simulink model "train_detection"  (R2024b)
settings: Solver=FixedStepAuto  StartTime=0.0  StopTime=simDuration  FixedStep=0.01  RelTol=1e-3
InitFcn:
  | breakp=[-1, -0.9, -0.8, -0.6, -0.4, -0.2, -0.1, 0, 0.1, 0.2, 0.4, 0.6, 0.8, 1];
  | 
  | splinenew =[-1, -0.92, -0.8, -0.50, -0.28, -0.12, -0.05, 0, 0.005, 0.01, 0.02, 0.025,0.03,0.035];
undefined symbols (not defined in the file or in its folder): Discrete, K, qbreak, Time
libraries: simulink x25, ctrlSharedLib x4, dspfdesign x2
(part 1 of 2)
settings Model: Creator=ARIES  LastModifiedBy=zglin

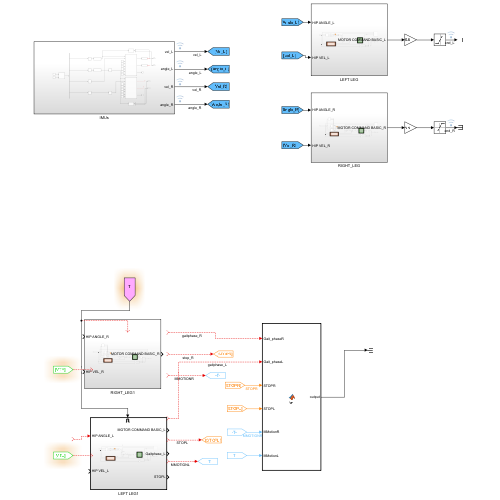
[thumbnail: Simulink's stored preview of the top-level diagram]
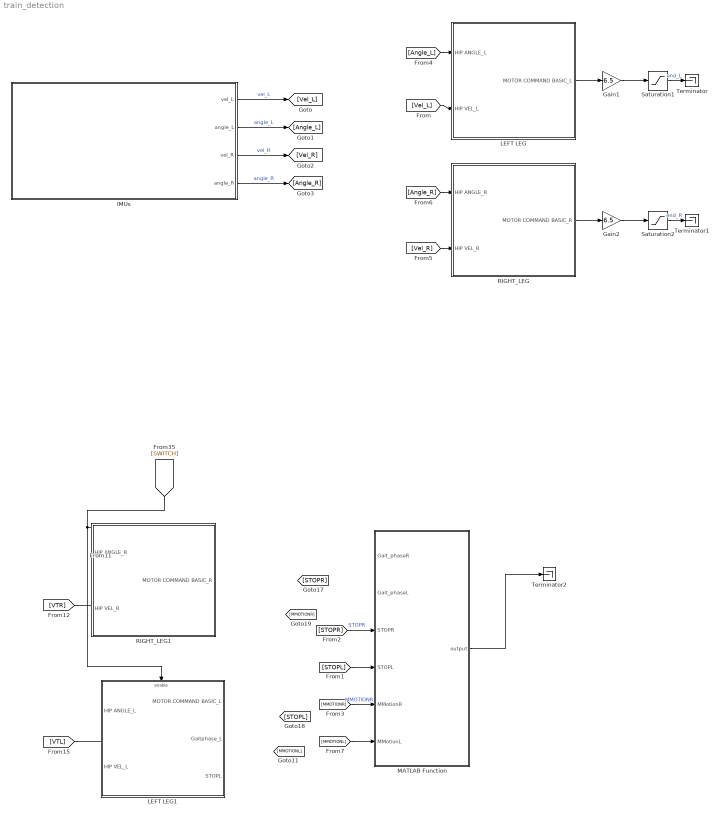
== system train_detection ==
  Gain1 : Gain  Gain=6.5
  Gain2 : Gain  Gain=6.5
  IMUs : Subsystem
  LEFT LEG : Subsystem
  LEFT LEG1 : Subsystem
  MATLAB Function : MATLAB Function  TreatAsAtomicUnit=on
  RIGHT_LEG : Subsystem
  RIGHT_LEG1 : Subsystem
  Saturation1 : Saturate  UpperLimit=900*pi/180  LowerLimit=-900*pi/180
  Saturation2 : Saturate  UpperLimit=900*pi/180  LowerLimit=-900*pi/180
  Terminator : Terminator
  Terminator1 : Terminator
  Terminator2 : Terminator
  wires:
  IMUs/1(vel_L) -> [Vel_L]  "vel_L"
  IMUs/3(vel_R) -> [Vel_R]  "vel_R"
  IMUs/4(angle_R) -> [Angle_R]  "angle_R"
  IMUs/2(angle_L) -> [Angle_L]  "angle_L"
  [Angle_R] -> RIGHT_LEG/1(HIP ANGLE_R)
  RIGHT_LEG/1(MOTOR COMMAND BASIC_R) -> Gain2/1
  [Vel_L] -> LEFT LEG/2(HIP VEL_L)
  [Vel_R] -> RIGHT_LEG/2(HIP VEL_R)
  [Angle_L] -> LEFT LEG/1(HIP ANGLE_L)
  LEFT LEG/1(MOTOR COMMAND BASIC_L) -> Gain1/1
  Gain1/1 -> Saturation1/1
  Gain2/1 -> Saturation2/1
  Saturation1/1 -> Terminator/1  "end_L"
  Saturation2/1 -> Terminator1/1  "end_R"
  ? -> LEFT LEG1/1(HIP ANGLE_L)
  ? -> [STOPR]  "stop_R"
  ? -> [STOPL]  "STOPL"
  [MMOTIONR] -> MATLAB Function/5(MMotionR)  "MMOTIONR"
  [STOPL] -> MATLAB Function/4(STOPL)
  ? -> [MMOTIONL]  "MMOTIONL"
  [MMOTIONL] -> MATLAB Function/6(MMotionL)
  MATLAB Function/1(output) -> Terminator2/1
  ? -> [MMOTIONR]  "MMOTIONR"
  ? -> MATLAB Function/2(Gait_phaseL)  "gaitphase_L"
  [VTL] -> ?
  [SWITCH] -> LEFT LEG1/Enable
  [VTR] -> ?
  ? -> MATLAB Function/1(Gait_phaseR)  "gaitphase_R"
  [STOPR] -> MATLAB Function/3(STOPR)  "STOPR"

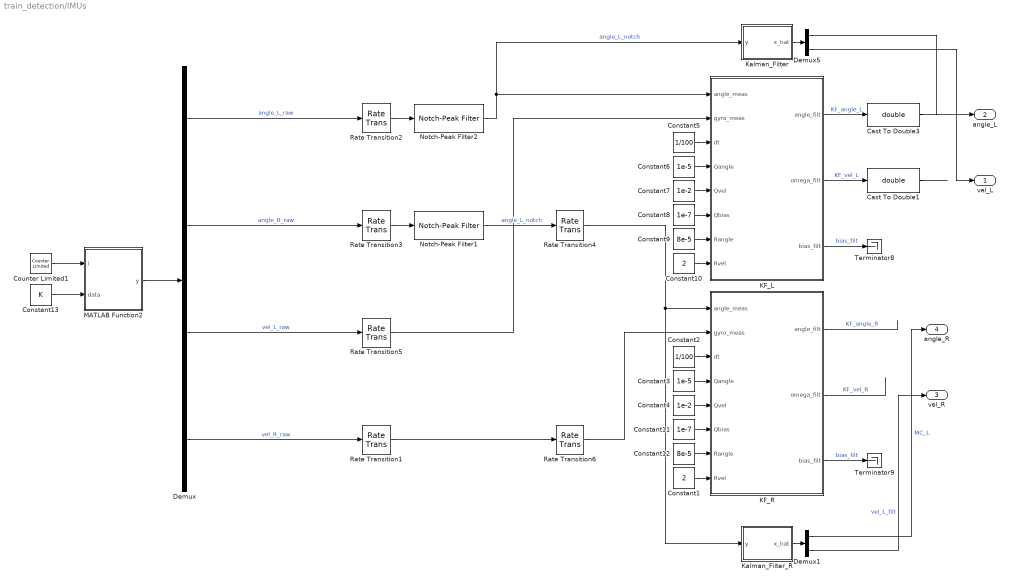
== system train_detection/IMUs ==
  Cast To Double1 : DataTypeConversion  OutDataTypeStr=double  SaturateOnIntegerOverflow=off  RndMeth=Floor
  Cast To Double3 : DataTypeConversion  OutDataTypeStr=double  SaturateOnIntegerOverflow=off  RndMeth=Floor
  Constant1 : Constant  Value=2
  Constant10 : Constant  Value=2
  Constant11 : Constant  Value=1e-7
  Constant12 : Constant  Value=8e-5
  Constant13 : Constant  Value=K
  Constant2 : Constant  Value=1/100
  Constant3 : Constant  Value=1e-5
  Constant4 : Constant  Value=1e-2
  Constant5 : Constant  Value=1/100
  Constant6 : Constant  Value=1e-5
  Constant7 : Constant  Value=1e-2
  Constant8 : Constant  Value=1e-7
  Constant9 : Constant  Value=8e-5
  Counter Limited1 : simulink/Sources/Counter Limited  uplimit=size(K,1)  tsamp=0.01
  Demux : Demux
  Demux1 : Demux  Outputs=2
  Demux5 : Demux  Outputs=2
  KF_L : MATLAB Function  TreatAsAtomicUnit=on  SystemSampleTime=0.01
  KF_R : MATLAB Function  TreatAsAtomicUnit=on  SystemSampleTime=0.01
  Kalman_Filter : MATLAB Function  TreatAsAtomicUnit=on
  Kalman_Filter_R : MATLAB Function  TreatAsAtomicUnit=on
  MATLAB Function2 : MATLAB Function  TreatAsAtomicUnit=on
  Notch-Peak Filter1 : dspfdesign/Notch-Peak Filter  Specification=Bandwidth and center frequency  BandwidthPort=off  Bandwidth=0.1  QualityFactorPort=off  QualityFactor=5  CenterFrequencyPort=off  CenterFrequency=0  BandwidthCoefficientPort=off  BandwidthCoefficient=0.72654  CenterFrequencyCoefficientPort=off  CenterFrequencyCoefficient=0  Output=Notch  SampleRateMode=Specify on dialog  SampleRate=100  SimulateUsing=Interpreted execution
  Notch-Peak Filter2 : dspfdesign/Notch-Peak Filter  Specification=Bandwidth and center frequency  BandwidthPort=off  Bandwidth=0.1  QualityFactorPort=off  QualityFactor=5  CenterFrequencyPort=off  CenterFrequency=0  BandwidthCoefficientPort=off  BandwidthCoefficient=0.72654  CenterFrequencyCoefficientPort=off  CenterFrequencyCoefficient=0  Output=Notch  SampleRateMode=Specify on dialog  SampleRate=100  SimulateUsing=Interpreted execution
  Rate Transition{1..6} (6 alike) : RateTransition  OutPortSampleTime=0.01
  Terminator8 : Terminator
  Terminator9 : Terminator
  vel_L : Outport
  angle_L : Outport  Port=2
  vel_R : Outport  Port=3
  angle_R : Outport  Port=4
  wires:
  Constant1/1 -> KF_R/8(Rvel)
  Counter Limited1/1 -> MATLAB Function2/1(i)
  MATLAB Function2/1(y) -> Demux/1
  Demux5/2 -> vel_L/1
  Demux/1 -> Rate Transition2/1  "angle_L_raw"
  Demux5/1 -> angle_L/1
  Rate Transition6/1 -> KF_R/2(gyro_meas)
  Constant6/1 -> KF_L/4(Qangle)
  Constant13/1 -> MATLAB Function2/2(data)
  Demux/4 -> Rate Transition1/1  "vel_R_raw"
  Rate Transition5/1 -> KF_L/2(gyro_meas)
  Demux1/1 -> angle_R/1  "MC_L"
  Demux1/2 -> vel_R/1  "vel_L_filt"
  Notch-Peak Filter1/1 -> Rate Transition4/1  "angle_L_notch"
  Constant10/1 -> KF_L/8(Rvel)
  KF_L/2(omega_filt) -> Cast To Double1/1  "KF_vel_L"
  Rate Transition1/1 -> Rate Transition6/1
  Constant5/1 -> KF_L/3(dt)
  Rate Transition3/1 -> Notch-Peak Filter1/1
  Constant8/1 -> KF_L/6(Qbias)
  Constant3/1 -> KF_R/4(Qangle)
  KF_L/3(bias_filt) -> Terminator8/1  "bias_filt"
  Demux/3 -> Rate Transition5/1  "vel_L_raw"
  Constant2/1 -> KF_R/3(dt)
  KF_R/3(bias_filt) -> Terminator9/1  "bias_filt"
  Demux/2 -> Rate Transition3/1  "angle_R_raw"
  Constant11/1 -> KF_R/6(Qbias)
  KF_L/1(angle_filt) -> Cast To Double3/1  "KF_angle_L"
  Constant12/1 -> KF_R/7(Rangle)
  Constant9/1 -> KF_L/7(Rangle)
  Constant7/1 -> KF_L/5(Qvel)
  Constant4/1 -> KF_R/5(Qvel)
  Rate Transition2/1 -> Notch-Peak Filter2/1
  Rate Transition4/1 -> KF_R/1(angle_meas), Kalman_Filter_R/1(y)
  Kalman_Filter/1(x_hat) -> Demux5/1
  Kalman_Filter_R/1(x_hat) -> Demux1/1
  Notch-Peak Filter2/1 -> Kalman_Filter/1(y), KF_L/1(angle_meas)  "angle_L_notch"
  KF_R/1(angle_filt) -> ?  "KF_angle_R"
  KF_R/2(omega_filt) -> ?  "KF_vel_R"
  Cast To Double1/1 -> ?
  Cast To Double3/1 -> ?

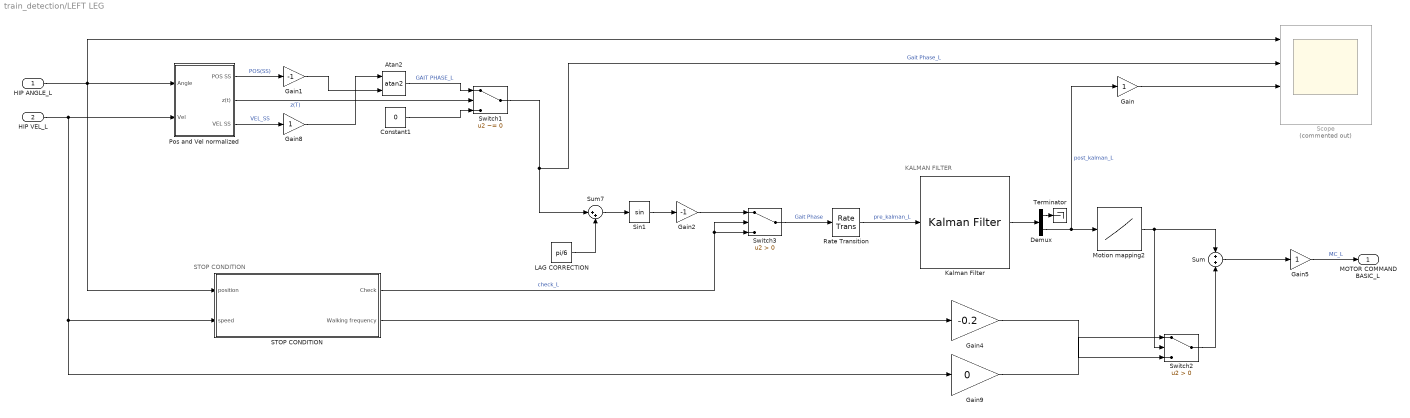
== system train_detection/LEFT LEG ==
  note: STOP CONDITION
  note: KALMAN FILTER
  HIP ANGLE_L : Inport
  HIP VEL_L : Inport  Port=2
  Atan2 : Trigonometry  Operator=atan2
  Constant1 : Constant  Value=0
  Demux : Demux  Outputs=2
  Gain : Gain
  Gain1 : Gain  Gain=-1
  Gain2 : Gain  Gain=-1
  Gain4 : Gain  Gain=-0.2
  Gain5 : Gain
  Gain8 : Gain
  Gain9 : Gain  Gain=0
  Kalman Filter : ctrlSharedLib/Kalman Filter  TimeDomain=Discrete-Time  UseCurrentEstimator=on  ModelSource=Individual A, B, C, D matrices  ModelSourceVariable=idss  A=[1 0.01;0 1]  B=eye(2)  C=[1 0]  D=zeros(2)  NumberOfStates=1  NumberOfInputs=1  NumberOfOutputs=1  InitialEstimateSource=Dialog  X0=0  P0=10  UseK=off  UseGH=off  NumberOfProcessNoiseInputs=2  G=1  TimeInvariantG=on  H=0  TimeInvariantH=on  Q=0.02  TimeInvariantQ=on  R=0.75  TimeInvariantR=on  N=0  TimeInvariantN=on  AddInputPort=off  AddEnablePort=off  OutputEstimatedY=off  OutputP=off  Ts=-1
  LAG CORRECTION : Constant  Value=pi/6
  Motion mapping2 : Lookup_n-D  NumberOfTableDimensions=1  BreakpointsForDimension1=breakp  BreakpointsForDimension2=qbreak(:,2)  Table=splinenew  InterpMethod=Cubic spline  ExtrapMethod=Cubic spline  InternalRulePriority=Speed  RndMeth=Simplest
  Pos and Vel normalized : Subsystem
  Rate Transition : RateTransition  OutPortSampleTime=0.01
  STOP CONDITION : Subsystem
  Scope : Scope  Commented=on  NumInputPorts=4
  Sin1 : Trigonometry
  Sum : Sum
  Sum7 : Sum  Inputs=|++
  Switch1 : Switch  Criteria=u2 ~= 0  SaturateOnIntegerOverflow=off  InputSameDT=off
  Switch2 : Switch  Criteria=u2 > Threshold  SaturateOnIntegerOverflow=off  InputSameDT=off
  Switch3 : Switch  Criteria=u2 > Threshold  SaturateOnIntegerOverflow=off  InputSameDT=off
  Terminator : Terminator
  MOTOR COMMAND BASIC_L : Outport
  wires:
  Kalman Filter/1 -> Demux/1
  Gain8/1 -> Atan2/1
  Gain2/1 -> Switch3/1
  STOP CONDITION/1(Check) -> Switch3/2, Switch3/3  "check_L"
  Rate Transition/1 -> Kalman Filter/1  "pre_kalman_L"
  Atan2/1 -> Switch1/1  "GAIT PHASE_L"
  Sin1/1 -> Gain2/1
  Switch1/1 -> Sum7/1, Scope/2  "Gait Phase_L"
  Switch3/1 -> Rate Transition/1  "Gait Phase"
  Constant1/1 -> Switch1/3
  Motion mapping2/1 -> Sum/1, Switch2/2
  Demux/1 -> Terminator/1
  LAG CORRECTION/1 -> Sum7/2
  Sum7/1 -> Sin1/1
  Gain1/1 -> Atan2/2
  Gain9/1 -> Switch2/1
  Gain4/1 -> Switch2/3
  Switch2/1 -> Sum/2
  Pos and Vel normalized/1(POS SS) -> Gain1/1  "POS(SS)"
  Pos and Vel normalized/2(z(t)) -> Switch1/2  "z(T)"
  Pos and Vel normalized/3(VEL SS) -> Gain8/1  "VEL_SS"
  Gain/1 -> Scope/3
  Demux/2 -> Gain/1, Motion mapping2/1  "post_kalman_L"
  Sum/1 -> Gain5/1
  STOP CONDITION/2(Walking frequency) -> Gain4/1
  Gain5/1 -> MOTOR COMMAND BASIC_L/1  "MC_L"
  HIP VEL_L/1 -> Pos and Vel normalized/2(Vel), STOP CONDITION/2(speed), Gain9/1
  HIP ANGLE_L/1 -> Pos and Vel normalized/1(Angle), Scope/1, STOP CONDITION/1(position)

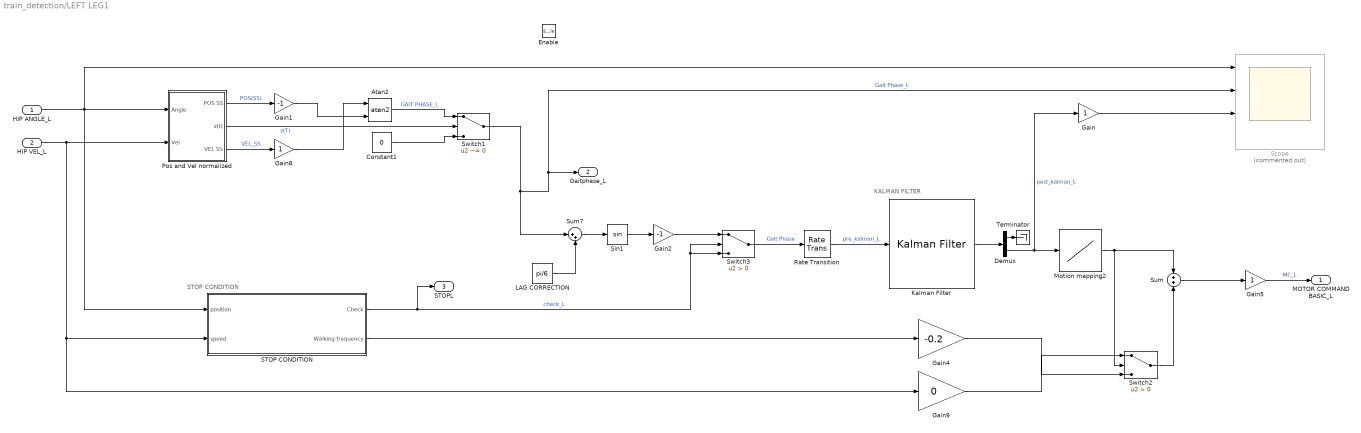
== system train_detection/LEFT LEG1 ==
  note: STOP CONDITION
  note: KALMAN FILTER
  HIP ANGLE_L : Inport
  HIP VEL_L : Inport  Port=2
  Enable : EnablePort
  Atan2 : Trigonometry  Operator=atan2
  Constant1 : Constant  Value=0
  Demux : Demux  Outputs=2
  Gain : Gain
  Gain1 : Gain  Gain=-1
  Gain2 : Gain  Gain=-1
  Gain4 : Gain  Gain=-0.2
  Gain5 : Gain
  Gain8 : Gain
  Gain9 : Gain  Gain=0
  Kalman Filter : ctrlSharedLib/Kalman Filter  TimeDomain=Discrete-Time  UseCurrentEstimator=on  ModelSource=Individual A, B, C, D matrices  ModelSourceVariable=idss  A=[1 0.01;0 1]  B=eye(2)  C=[1 0]  D=zeros(2)  NumberOfStates=1  NumberOfInputs=1  NumberOfOutputs=1  InitialEstimateSource=Dialog  X0=0  P0=10  UseK=off  UseGH=off  NumberOfProcessNoiseInputs=2  G=1  TimeInvariantG=on  H=0  TimeInvariantH=on  Q=0.02  TimeInvariantQ=on  R=0.75  TimeInvariantR=on  N=0  TimeInvariantN=on  AddInputPort=off  AddEnablePort=off  OutputEstimatedY=off  OutputP=off  Ts=-1
  LAG CORRECTION : Constant  Value=pi/6
  Motion mapping2 : Lookup_n-D  NumberOfTableDimensions=1  BreakpointsForDimension1=breakp  BreakpointsForDimension2=qbreak(:,2)  Table=splinenew  InterpMethod=Cubic spline  ExtrapMethod=Cubic spline  InternalRulePriority=Speed  RndMeth=Simplest
  Pos and Vel normalized : Subsystem
  Rate Transition : RateTransition  OutPortSampleTime=0.01
  STOP CONDITION : Subsystem
  Scope : Scope  Commented=on  NumInputPorts=4
  Sin1 : Trigonometry
  Sum : Sum
  Sum7 : Sum  Inputs=|++
  Switch1 : Switch  Criteria=u2 ~= 0  SaturateOnIntegerOverflow=off  InputSameDT=off
  Switch2 : Switch  Criteria=u2 > Threshold  SaturateOnIntegerOverflow=off  InputSameDT=off
  Switch3 : Switch  Criteria=u2 > Threshold  SaturateOnIntegerOverflow=off  InputSameDT=off
  Terminator : Terminator
  MOTOR COMMAND BASIC_L : Outport
  Gaitphase_L : Outport  Port=2
  STOPL : Outport  Port=3
  wires:
  Kalman Filter/1 -> Demux/1
  Gain8/1 -> Atan2/1
  Gain2/1 -> Switch3/1
  STOP CONDITION/1(Check) -> STOPL/1, Switch3/2, Switch3/3  "check_L"
  Rate Transition/1 -> Kalman Filter/1  "pre_kalman_L"
  Atan2/1 -> Switch1/1  "GAIT PHASE_L"
  Sin1/1 -> Gain2/1
  Switch1/1 -> Sum7/1, Gaitphase_L/1, Scope/2  "Gait Phase_L"
  Switch3/1 -> Rate Transition/1  "Gait Phase"
  Constant1/1 -> Switch1/3
  Motion mapping2/1 -> Sum/1, Switch2/2
  Demux/1 -> Terminator/1
  LAG CORRECTION/1 -> Sum7/2
  Sum7/1 -> Sin1/1
  Gain1/1 -> Atan2/2
  Gain9/1 -> Switch2/1
  Gain4/1 -> Switch2/3
  Switch2/1 -> Sum/2
  Pos and Vel normalized/1(POS SS) -> Gain1/1  "POS(SS)"
  Pos and Vel normalized/2(z(t)) -> Switch1/2  "z(T)"
  Pos and Vel normalized/3(VEL SS) -> Gain8/1  "VEL_SS"
  Gain/1 -> Scope/3
  Demux/2 -> Gain/1, Motion mapping2/1  "post_kalman_L"
  Sum/1 -> Gain5/1
  STOP CONDITION/2(Walking frequency) -> Gain4/1
  Gain5/1 -> MOTOR COMMAND BASIC_L/1  "MC_L"
  HIP VEL_L/1 -> Pos and Vel normalized/2(Vel), STOP CONDITION/2(speed), Gain9/1
  HIP ANGLE_L/1 -> Pos and Vel normalized/1(Angle), Scope/1, STOP CONDITION/1(position)

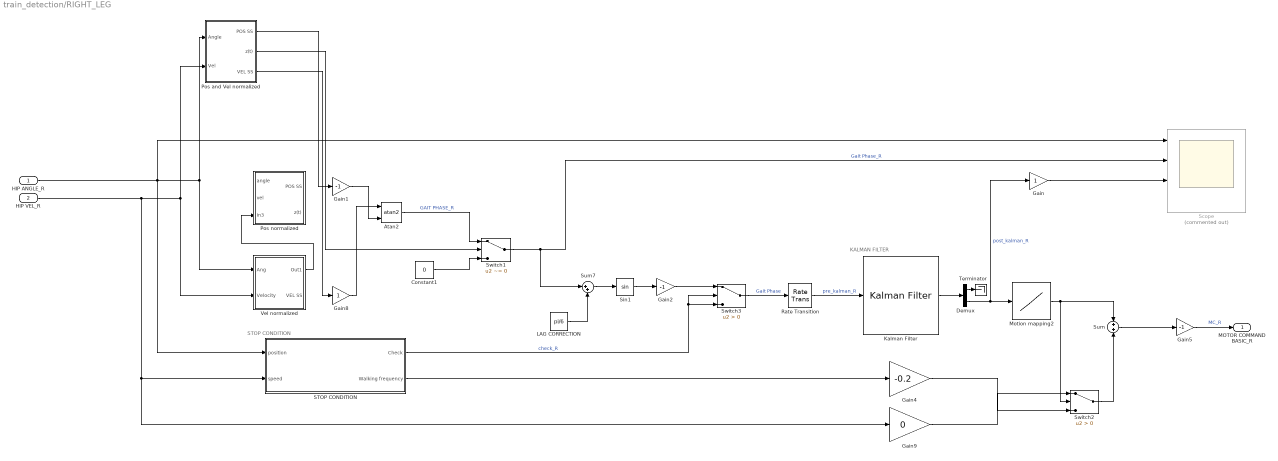
== system train_detection/RIGHT_LEG ==
  note: STOP CONDITION
  note: KALMAN FILTER
  HIP ANGLE_R : Inport
  HIP VEL_R : Inport  Port=2
  Atan2 : Trigonometry  Operator=atan2
  Constant1 : Constant  Value=0
  Demux : Demux  Outputs=2
  Gain : Gain
  Gain1 : Gain  Gain=-1
  Gain2 : Gain  Gain=-1
  Gain4 : Gain  Gain=-0.2
  Gain5 : Gain  Gain=-1
  Gain8 : Gain
  Gain9 : Gain  Gain=0
  Kalman Filter : ctrlSharedLib/Kalman Filter  TimeDomain=Discrete-Time  UseCurrentEstimator=on  ModelSource=Individual A, B, C, D matrices  ModelSourceVariable=idss  A=[1 0.01;0 1]  B=eye(2)  C=[1 0]  D=zeros(2)  NumberOfStates=1  NumberOfInputs=1  NumberOfOutputs=1  InitialEstimateSource=Dialog  X0=0  P0=10  UseK=off  UseGH=off  NumberOfProcessNoiseInputs=2  G=1  TimeInvariantG=on  H=0  TimeInvariantH=on  Q=0.02  TimeInvariantQ=on  R=0.75  TimeInvariantR=on  N=0  TimeInvariantN=on  AddInputPort=off  AddEnablePort=off  OutputEstimatedY=off  OutputP=off  Ts=-1
  LAG CORRECTION : Constant  Value=pi/6
  Motion mapping2 : Lookup_n-D  NumberOfTableDimensions=1  BreakpointsForDimension1=breakp  BreakpointsForDimension2=qbreak(:,2)  Table=splinenew  InterpMethod=Cubic spline  ExtrapMethod=Cubic spline  InternalRulePriority=Speed  RndMeth=Simplest
  Pos and Vel normalized : Subsystem
  Pos normalized : Subsystem
  Rate Transition : RateTransition  OutPortSampleTime=0.01
  STOP CONDITION : Subsystem
  Scope : Scope  Commented=on  NumInputPorts=4
  Sin1 : Trigonometry
  Sum : Sum
  Sum7 : Sum  Inputs=|++
  Switch1 : Switch  Criteria=u2 ~= 0  SaturateOnIntegerOverflow=off  InputSameDT=off
  Switch2 : Switch  Criteria=u2 > Threshold  SaturateOnIntegerOverflow=off  InputSameDT=off
  Switch3 : Switch  Criteria=u2 > Threshold  SaturateOnIntegerOverflow=off  InputSameDT=off
  Terminator : Terminator
  Vel normalized : Subsystem
  MOTOR COMMAND BASIC_R : Outport
  wires:
  Kalman Filter/1 -> Demux/1
  Gain8/1 -> Atan2/1
  Gain2/1 -> Switch3/1
  STOP CONDITION/1(Check) -> Switch3/2, Switch3/3  "check_R"
  Rate Transition/1 -> Kalman Filter/1  "pre_kalman_R"
  Atan2/1 -> Switch1/1  "GAIT PHASE_R"
  Sin1/1 -> Gain2/1
  Switch1/1 -> Sum7/1, Scope/2  "Gait Phase_R"
  HIP VEL_R/1 -> Pos and Vel normalized/2(Vel), Vel normalized/2(Velocity), STOP CONDITION/2(speed), Gain9/1
  Switch3/1 -> Rate Transition/1  "Gait Phase"
  Constant1/1 -> Switch1/3
  Motion mapping2/1 -> Sum/1, Switch2/2
  Demux/1 -> Terminator/1
  LAG CORRECTION/1 -> Sum7/2
  Sum7/1 -> Sin1/1
  Gain1/1 -> Atan2/2
  Gain9/1 -> Switch2/1
  Gain4/1 -> Switch2/3
  Switch2/1 -> Sum/2
  Pos and Vel normalized/1(POS SS) -> Gain1/1
  Pos and Vel normalized/2(z(t)) -> Switch1/2
  Vel normalized/1(Out1) -> Pos normalized/3(In3)
  Pos and Vel normalized/3(VEL SS) -> Gain8/1
  Gain/1 -> Scope/3
  HIP ANGLE_R/1 -> Scope/1, STOP CONDITION/1(position), Pos and Vel normalized/1(Angle), Vel normalized/1(Ang)
  Demux/2 -> Gain/1, Motion mapping2/1  "post_kalman_R"
  Sum/1 -> Gain5/1
  STOP CONDITION/2(Walking frequency) -> Gain4/1
  Gain5/1 -> MOTOR COMMAND BASIC_R/1  "MC_R"

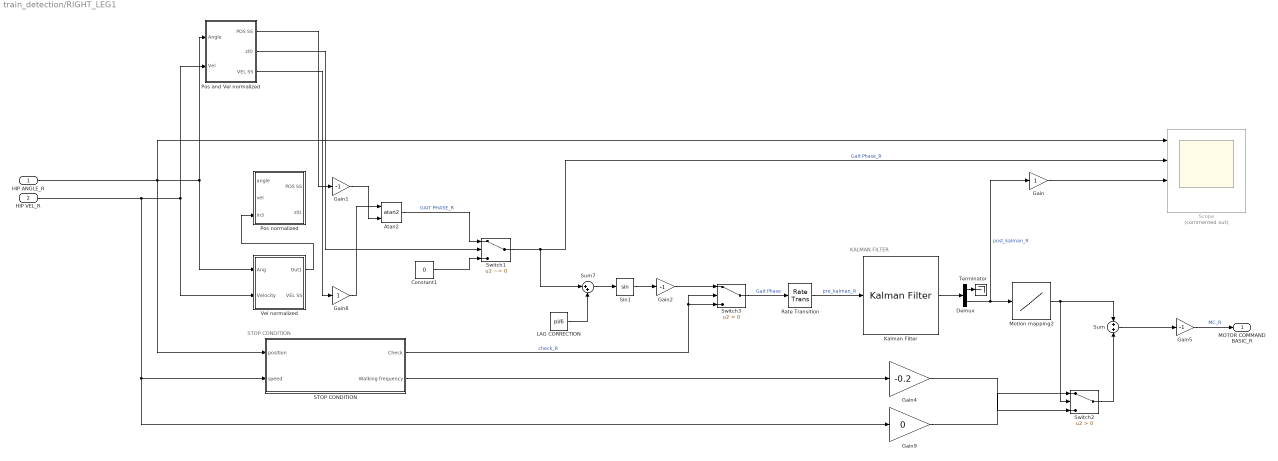
== system train_detection/RIGHT_LEG1 ==
  note: STOP CONDITION
  note: KALMAN FILTER
  HIP ANGLE_R : Inport
  HIP VEL_R : Inport  Port=2
  Atan2 : Trigonometry  Operator=atan2
  Constant1 : Constant  Value=0
  Demux : Demux  Outputs=2
  Gain : Gain
  Gain1 : Gain  Gain=-1
  Gain2 : Gain  Gain=-1
  Gain4 : Gain  Gain=-0.2
  Gain5 : Gain  Gain=-1
  Gain8 : Gain
  Gain9 : Gain  Gain=0
  Kalman Filter : ctrlSharedLib/Kalman Filter  TimeDomain=Discrete-Time  UseCurrentEstimator=on  ModelSource=Individual A, B, C, D matrices  ModelSourceVariable=idss  A=[1 0.01;0 1]  B=eye(2)  C=[1 0]  D=zeros(2)  NumberOfStates=1  NumberOfInputs=1  NumberOfOutputs=1  InitialEstimateSource=Dialog  X0=0  P0=10  UseK=off  UseGH=off  NumberOfProcessNoiseInputs=2  G=1  TimeInvariantG=on  H=0  TimeInvariantH=on  Q=0.02  TimeInvariantQ=on  R=0.75  TimeInvariantR=on  N=0  TimeInvariantN=on  AddInputPort=off  AddEnablePort=off  OutputEstimatedY=off  OutputP=off  Ts=-1
  LAG CORRECTION : Constant  Value=pi/6
  Motion mapping2 : Lookup_n-D  NumberOfTableDimensions=1  BreakpointsForDimension1=breakp  BreakpointsForDimension2=qbreak(:,2)  Table=splinenew  InterpMethod=Cubic spline  ExtrapMethod=Cubic spline  InternalRulePriority=Speed  RndMeth=Simplest
  Pos and Vel normalized : Subsystem
  Pos normalized : Subsystem
  Rate Transition : RateTransition  OutPortSampleTime=0.01
  STOP CONDITION : Subsystem
  Scope : Scope  Commented=on  NumInputPorts=4
  Sin1 : Trigonometry
  Sum : Sum
  Sum7 : Sum  Inputs=|++
  Switch1 : Switch  Criteria=u2 ~= 0  SaturateOnIntegerOverflow=off  InputSameDT=off
  Switch2 : Switch  Criteria=u2 > Threshold  SaturateOnIntegerOverflow=off  InputSameDT=off
  Switch3 : Switch  Criteria=u2 > Threshold  SaturateOnIntegerOverflow=off  InputSameDT=off
  Terminator : Terminator
  Vel normalized : Subsystem
  MOTOR COMMAND BASIC_R : Outport
  wires:
  Kalman Filter/1 -> Demux/1
  Gain8/1 -> Atan2/1
  Gain2/1 -> Switch3/1
  STOP CONDITION/1(Check) -> Switch3/2, Switch3/3  "check_R"
  Rate Transition/1 -> Kalman Filter/1  "pre_kalman_R"
  Atan2/1 -> Switch1/1  "GAIT PHASE_R"
  Sin1/1 -> Gain2/1
  Switch1/1 -> Sum7/1, Scope/2  "Gait Phase_R"
  HIP VEL_R/1 -> Pos and Vel normalized/2(Vel), Vel normalized/2(Velocity), STOP CONDITION/2(speed), Gain9/1
  Switch3/1 -> Rate Transition/1  "Gait Phase"
  Constant1/1 -> Switch1/3
  Motion mapping2/1 -> Sum/1, Switch2/2
  Demux/1 -> Terminator/1
  LAG CORRECTION/1 -> Sum7/2
  Sum7/1 -> Sin1/1
  Gain1/1 -> Atan2/2
  Gain9/1 -> Switch2/1
  Gain4/1 -> Switch2/3
  Switch2/1 -> Sum/2
  Pos and Vel normalized/1(POS SS) -> Gain1/1
  Pos and Vel normalized/2(z(t)) -> Switch1/2
  Vel normalized/1(Out1) -> Pos normalized/3(In3)
  Pos and Vel normalized/3(VEL SS) -> Gain8/1
  Gain/1 -> Scope/3
  HIP ANGLE_R/1 -> Scope/1, STOP CONDITION/1(position), Pos and Vel normalized/1(Angle), Vel normalized/1(Ang)
  Demux/2 -> Gain/1, Motion mapping2/1  "post_kalman_R"
  Sum/1 -> Gain5/1
  STOP CONDITION/2(Walking frequency) -> Gain4/1
  Gain5/1 -> MOTOR COMMAND BASIC_R/1  "MC_R"

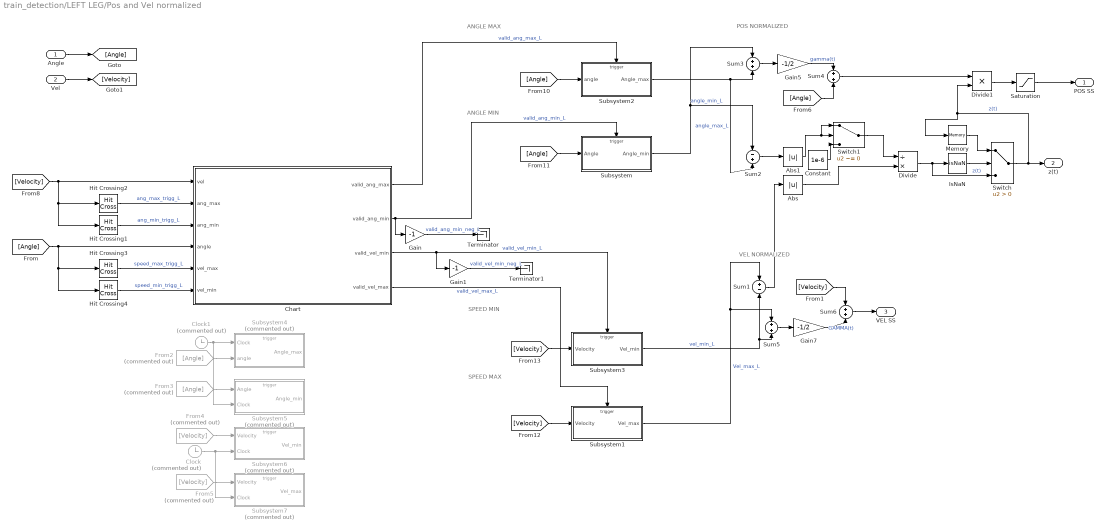
== system train_detection/LEFT LEG/Pos and Vel normalized ==
  note: ANGLE MIN
  note: ANGLE MAX
  note: SPEED MAX
  note: SPEED MIN
  note: POS NORMALIZED
  note: VEL NORMALIZED
  Angle : Inport
  Vel : Inport  Port=2
  Abs : Abs  SaturateOnIntegerOverflow=off
  Abs1 : Abs  SaturateOnIntegerOverflow=off
  Chart : Stateflow chart  TreatAsAtomicUnit=on
      settings: PortSchema="{\"entries\":[{\"content\":{\"sides\":[{\"content\":{\"connectorIds\":[\"In5\",\"In1\",\"In4\",\"In6\",\"In3\",\"In2\"]},\"type\":\"ConnectorPlacement.EquallySpacedRectSide\",\"uuid\":\"1b4e9464-0c1b-4aef-9691-eb83c0a92a72\"},{\"content\":{\"connectorIds\":[\"Out3\",\"Out4\",\"Out2\",\"Out1\"],\"side\":\"RIGHT\"},\"type\":\"ConnectorPlacement.EquallySpacedRectSide\",\"uuid\":\"791196f6-4c97-40a1-8015-a03f83b94293\"},{\"content\":{\"side\":\"TOP\"},\"type\":\"ConnectorPlacement.EquallySpacedRectSide\",\"uuid\":\"116d3fb6-be2c-4be4-86cc-df9779b501c6\"}]},\"type\":\"ConnectorPlacement.EquallySpacedConnector\",\"uuid\":\"13d090b2-a2d1-429a-b321-7320a6f027c7\"}],\"packageUris\":[\"http://schema.mathworks.com/mf0/Connector/R2020b\"],\"version\":\"1.0\"}"
  Clock : Clock  Commented=on
  Clock1 : Clock  Commented=on
  Constant : Constant  Value=1e-6
  Divide : Product  Inputs=/*
  Divide1 : Product  Inputs=**
  From2 : From  Commented=on  GotoTag=Angle
  From3 : From  Commented=on  GotoTag=Angle
  From4 : From  Commented=on  GotoTag=Velocity
  From5 : From  Commented=on  GotoTag=Velocity
  Gain : Gain  Gain=-1
  Gain1 : Gain  Gain=-1
  Gain5 : Gain  Gain=-1/2
  Gain7 : Gain  Gain=-1/2
  Hit Crossing1 : HitCross  HitCrossingDirection=rising
  Hit Crossing2 : HitCross  HitCrossingDirection=falling
  Hit Crossing3 : HitCross  HitCrossingDirection=rising
  Hit Crossing4 : HitCross  HitCrossingDirection=falling
  IsNaN : RelationalOperator  Operator=isNaN  OutDataTypeStr=boolean  RndMeth=Simplest  InputSameDT=off
  Memory : Memory
  Saturation : Saturate  UpperLimit=10  LowerLimit=-10
  Subsystem : Subsystem
  Subsystem1 : Subsystem
  Subsystem2 : Subsystem
  Subsystem3 : Subsystem
  Subsystem4 : Subsystem  Commented=on
  Subsystem5 : Subsystem  Commented=on
  Subsystem6 : Subsystem  Commented=on
  Subsystem7 : Subsystem  Commented=on
  Sum1 : Sum  Inputs=+-
  Sum2 : Sum  Inputs=-+
  Sum{3..6} (4 alike) : Sum
  Switch : Switch  Criteria=u2 > Threshold  SaturateOnIntegerOverflow=off  InputSameDT=off
  Switch1 : Switch  Criteria=u2 ~= 0  SaturateOnIntegerOverflow=off  InputSameDT=off
  Terminator : Terminator
  Terminator1 : Terminator
  POS SS : Outport
  z(t) : Outport  Port=2
  VEL SS : Outport  Port=3
  wires:
  Hit Crossing2/1 -> Chart/1(ang_max)  "ang_max_trigg_L"
  Subsystem2/1(Angle_max) -> Sum2/2, Sum3/2  "angle_max_L"
  Sum4/1 -> Divide1/1
  Sum3/1 -> Gain5/1
  Subsystem/1(Angle_min) -> Sum2/1, Sum3/1  "angle_min_L"
  Hit Crossing1/1 -> Chart/4(ang_min)  "ang_min_trigg_L"
  Sum2/1 -> Abs1/1
  Sum1/1 -> Abs/1
  Gain5/1 -> Sum4/1  "gamma(t)"
  Abs/1 -> Divide/2
  Divide/1 -> IsNaN/1, Switch/3  "z(t)"
  Memory/1 -> Switch/1
  IsNaN/1 -> Switch/2
  Switch/1 -> Memory/1, Divide1/2, z(t)/1  "z(t)"
  Divide1/1 -> Saturation/1
  Saturation/1 -> POS SS/1
  Clock1/1 -> Subsystem5/2(Clock), Subsystem4/1(Clock)
  Constant/1 -> Switch1/3
  Abs1/1 -> Switch1/2, Switch1/1
  Switch1/1 -> Divide/1
  Clock/1 -> Subsystem7/2(Clock), Subsystem6/2(Clock)
  Hit Crossing4/1 -> Chart/2(vel_min)  "speed_min_trigg_L"
  Subsystem3/1(Vel_min) -> Sum1/2, Sum5/2  "vel_min_L"
  Subsystem1/1(Vel_max) -> Sum1/1, Sum5/1  "Vel_max_L"
  Sum5/1 -> Gain7/1
  Hit Crossing3/1 -> Chart/3(vel_max)  "speed_max_trigg_L"
  Sum6/1 -> VEL SS/1
  Gain7/1 -> Sum6/2  "GAMMA(t)"
  [Velocity] -> Sum6/1
  Chart/1(valid_vel_max) -> Subsystem1/Trigger  "valid_vel_max_L"
  Chart/4(valid_ang_min) -> Gain/1, Subsystem/Trigger  "valid_ang_min_L"
  Chart/3(valid_ang_max) -> Subsystem2/Trigger  "valid_ang_max_L"
  Chart/2(valid_vel_min) -> Gain1/1, Subsystem3/Trigger  "valid_vel_min_L"
  Vel/1 -> [Velocity]
  Angle/1 -> [Angle]
  From5/1 -> Subsystem7/1(Velocity)
  From4/1 -> Subsystem6/1(Velocity)
  From3/1 -> Subsystem5/1(Angle)
  From2/1 -> Subsystem4/2(angle)
  [Angle] -> Hit Crossing4/1, Hit Crossing3/1, Chart/6(angle)
  [Angle] -> Subsystem/1(Angle)
  [Angle] -> Subsystem2/1(angle)
  [Velocity] -> Subsystem1/1(Velocity)
  [Velocity] -> Subsystem3/1(Velocity)
  [Velocity] -> Hit Crossing1/1, Hit Crossing2/1, Chart/5(vel)
  Gain/1 -> Terminator/1  "valid_ang_min_neg_L"
  Gain1/1 -> Terminator1/1  "valid_vel_min_neg_L"
  [Angle] -> Sum4/2

== system train_detection/LEFT LEG/STOP CONDITION ==
  position : Inport
  speed : Inport  Port=2
  Constant : Constant
  Constant1 : Constant  Value=0
  Sqrt : Sqrt
  Square : Math  Operator=square
  Square1 : Math  Operator=square
  Sum : Sum
  Switch3 : Switch  Criteria=u2 > Threshold  Threshold=0.3  SaturateOnIntegerOverflow=off  InputSameDT=off
  Check : Outport
  Walking frequency : Outport  Port=2
  wires:
  position/1 -> Square/1  "θ"
  speed/1 -> Square1/1  "θ_dot"
  Square/1 -> Sum/1
  Square1/1 -> Sum/2
  Sum/1 -> Sqrt/1
  Constant/1 -> Switch3/1
  Constant1/1 -> Switch3/3
  Sqrt/1 -> Switch3/2, Walking frequency/1
  Switch3/1 -> Check/1

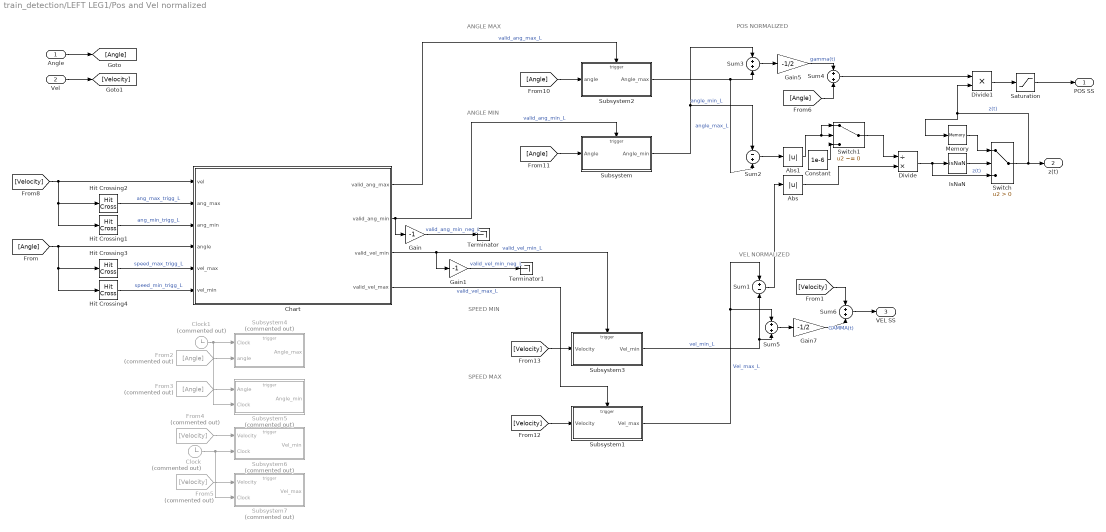
== system train_detection/LEFT LEG1/Pos and Vel normalized ==
  note: ANGLE MIN
  note: ANGLE MAX
  note: SPEED MAX
  note: SPEED MIN
  note: POS NORMALIZED
  note: VEL NORMALIZED
  Angle : Inport
  Vel : Inport  Port=2
  Abs : Abs  SaturateOnIntegerOverflow=off
  Abs1 : Abs  SaturateOnIntegerOverflow=off
  Chart : Stateflow chart  TreatAsAtomicUnit=on
      settings: PortSchema="{\"entries\":[{\"content\":{\"sides\":[{\"content\":{\"connectorIds\":[\"In5\",\"In1\",\"In4\",\"In6\",\"In3\",\"In2\"]},\"type\":\"ConnectorPlacement.EquallySpacedRectSide\",\"uuid\":\"1b4e9464-0c1b-4aef-9691-eb83c0a92a72\"},{\"content\":{\"connectorIds\":[\"Out3\",\"Out4\",\"Out2\",\"Out1\"],\"side\":\"RIGHT\"},\"type\":\"ConnectorPlacement.EquallySpacedRectSide\",\"uuid\":\"791196f6-4c97-40a1-8015-a03f83b94293\"},{\"content\":{\"side\":\"TOP\"},\"type\":\"ConnectorPlacement.EquallySpacedRectSide\",\"uuid\":\"116d3fb6-be2c-4be4-86cc-df9779b501c6\"}]},\"type\":\"ConnectorPlacement.EquallySpacedConnector\",\"uuid\":\"13d090b2-a2d1-429a-b321-7320a6f027c7\"}],\"packageUris\":[\"http://schema.mathworks.com/mf0/Connector/R2020b\"],\"version\":\"1.0\"}"
  Clock : Clock  Commented=on
  Clock1 : Clock  Commented=on
  Constant : Constant  Value=1e-6
  Divide : Product  Inputs=/*
  Divide1 : Product  Inputs=**
  From2 : From  Commented=on  GotoTag=Angle
  From3 : From  Commented=on  GotoTag=Angle
  From4 : From  Commented=on  GotoTag=Velocity
  From5 : From  Commented=on  GotoTag=Velocity
  Gain : Gain  Gain=-1
  Gain1 : Gain  Gain=-1
  Gain5 : Gain  Gain=-1/2
  Gain7 : Gain  Gain=-1/2
  Hit Crossing1 : HitCross  HitCrossingDirection=rising
  Hit Crossing2 : HitCross  HitCrossingDirection=falling
  Hit Crossing3 : HitCross  HitCrossingDirection=rising
  Hit Crossing4 : HitCross  HitCrossingDirection=falling
  IsNaN : RelationalOperator  Operator=isNaN  OutDataTypeStr=boolean  RndMeth=Simplest  InputSameDT=off
  Memory : Memory
  Saturation : Saturate  UpperLimit=10  LowerLimit=-10
  Subsystem : Subsystem
  Subsystem1 : Subsystem
  Subsystem2 : Subsystem
  Subsystem3 : Subsystem
  Subsystem4 : Subsystem  Commented=on
  Subsystem5 : Subsystem  Commented=on
  Subsystem6 : Subsystem  Commented=on
  Subsystem7 : Subsystem  Commented=on
  Sum1 : Sum  Inputs=+-
  Sum2 : Sum  Inputs=-+
  Sum{3..6} (4 alike) : Sum
  Switch : Switch  Criteria=u2 > Threshold  SaturateOnIntegerOverflow=off  InputSameDT=off
  Switch1 : Switch  Criteria=u2 ~= 0  SaturateOnIntegerOverflow=off  InputSameDT=off
  Terminator : Terminator
  Terminator1 : Terminator
  POS SS : Outport
  z(t) : Outport  Port=2
  VEL SS : Outport  Port=3
  wires:
  Hit Crossing2/1 -> Chart/1(ang_max)  "ang_max_trigg_L"
  Subsystem2/1(Angle_max) -> Sum2/2, Sum3/2  "angle_max_L"
  Sum4/1 -> Divide1/1
  Sum3/1 -> Gain5/1
  Subsystem/1(Angle_min) -> Sum2/1, Sum3/1  "angle_min_L"
  Hit Crossing1/1 -> Chart/4(ang_min)  "ang_min_trigg_L"
  Sum2/1 -> Abs1/1
  Sum1/1 -> Abs/1
  Gain5/1 -> Sum4/1  "gamma(t)"
  Abs/1 -> Divide/2
  Divide/1 -> IsNaN/1, Switch/3  "z(t)"
  Memory/1 -> Switch/1
  IsNaN/1 -> Switch/2
  Switch/1 -> Memory/1, Divide1/2, z(t)/1  "z(t)"
  Divide1/1 -> Saturation/1
  Saturation/1 -> POS SS/1
  Clock1/1 -> Subsystem5/2(Clock), Subsystem4/1(Clock)
  Constant/1 -> Switch1/3
  Abs1/1 -> Switch1/2, Switch1/1
  Switch1/1 -> Divide/1
  Clock/1 -> Subsystem7/2(Clock), Subsystem6/2(Clock)
  Hit Crossing4/1 -> Chart/2(vel_min)  "speed_min_trigg_L"
  Subsystem3/1(Vel_min) -> Sum1/2, Sum5/2  "vel_min_L"
  Subsystem1/1(Vel_max) -> Sum1/1, Sum5/1  "Vel_max_L"
  Sum5/1 -> Gain7/1
  Hit Crossing3/1 -> Chart/3(vel_max)  "speed_max_trigg_L"
  Sum6/1 -> VEL SS/1
  Gain7/1 -> Sum6/2  "GAMMA(t)"
  [Velocity] -> Sum6/1
  Chart/1(valid_vel_max) -> Subsystem1/Trigger  "valid_vel_max_L"
  Chart/4(valid_ang_min) -> Gain/1, Subsystem/Trigger  "valid_ang_min_L"
  Chart/3(valid_ang_max) -> Subsystem2/Trigger  "valid_ang_max_L"
  Chart/2(valid_vel_min) -> Gain1/1, Subsystem3/Trigger  "valid_vel_min_L"
  Vel/1 -> [Velocity]
  Angle/1 -> [Angle]
  From5/1 -> Subsystem7/1(Velocity)
  From4/1 -> Subsystem6/1(Velocity)
  From3/1 -> Subsystem5/1(Angle)
  From2/1 -> Subsystem4/2(angle)
  [Angle] -> Hit Crossing4/1, Hit Crossing3/1, Chart/6(angle)
  [Angle] -> Subsystem/1(Angle)
  [Angle] -> Subsystem2/1(angle)
  [Velocity] -> Subsystem1/1(Velocity)
  [Velocity] -> Subsystem3/1(Velocity)
  [Velocity] -> Hit Crossing1/1, Hit Crossing2/1, Chart/5(vel)
  Gain/1 -> Terminator/1  "valid_ang_min_neg_L"
  Gain1/1 -> Terminator1/1  "valid_vel_min_neg_L"
  [Angle] -> Sum4/2

== system train_detection/LEFT LEG1/STOP CONDITION ==
  position : Inport
  speed : Inport  Port=2
  Constant : Constant
  Constant1 : Constant  Value=0
  Sqrt : Sqrt
  Square : Math  Operator=square
  Square1 : Math  Operator=square
  Sum : Sum
  Switch3 : Switch  Criteria=u2 > Threshold  Threshold=0.3  SaturateOnIntegerOverflow=off  InputSameDT=off
  Check : Outport
  Walking frequency : Outport  Port=2
  wires:
  position/1 -> Square/1  "θ"
  speed/1 -> Square1/1  "θ_dot"
  Square/1 -> Sum/1
  Square1/1 -> Sum/2
  Sum/1 -> Sqrt/1
  Constant/1 -> Switch3/1
  Constant1/1 -> Switch3/3
  Sqrt/1 -> Switch3/2, Walking frequency/1
  Switch3/1 -> Check/1

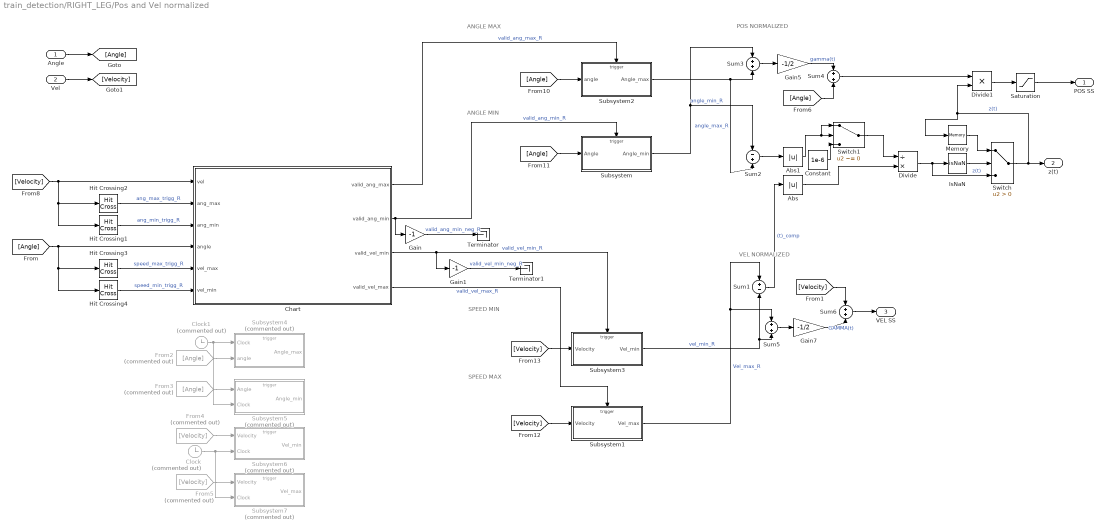
== system train_detection/RIGHT_LEG/Pos and Vel normalized ==
  note: ANGLE MIN
  note: ANGLE MAX
  note: SPEED MAX
  note: SPEED MIN
  note: POS NORMALIZED
  note: VEL NORMALIZED
  Angle : Inport
  Vel : Inport  Port=2
  Abs : Abs  SaturateOnIntegerOverflow=off
  Abs1 : Abs  SaturateOnIntegerOverflow=off
  Chart : Stateflow chart  TreatAsAtomicUnit=on
      settings: PortSchema="{\"entries\":[{\"content\":{\"sides\":[{\"content\":{\"connectorIds\":[\"In5\",\"In1\",\"In4\",\"In6\",\"In3\",\"In2\"]},\"type\":\"ConnectorPlacement.EquallySpacedRectSide\",\"uuid\":\"1b4e9464-0c1b-4aef-9691-eb83c0a92a72\"},{\"content\":{\"connectorIds\":[\"Out3\",\"Out4\",\"Out2\",\"Out1\"],\"side\":\"RIGHT\"},\"type\":\"ConnectorPlacement.EquallySpacedRectSide\",\"uuid\":\"791196f6-4c97-40a1-8015-a03f83b94293\"},{\"content\":{\"side\":\"TOP\"},\"type\":\"ConnectorPlacement.EquallySpacedRectSide\",\"uuid\":\"116d3fb6-be2c-4be4-86cc-df9779b501c6\"}]},\"type\":\"ConnectorPlacement.EquallySpacedConnector\",\"uuid\":\"13d090b2-a2d1-429a-b321-7320a6f027c7\"}],\"packageUris\":[\"http://schema.mathworks.com/mf0/Connector/R2020b\"],\"version\":\"1.0\"}"
  Clock : Clock  Commented=on
  Clock1 : Clock  Commented=on
  Constant : Constant  Value=1e-6
  Divide : Product  Inputs=/*
  Divide1 : Product  Inputs=**
  From2 : From  Commented=on  GotoTag=Angle
  From3 : From  Commented=on  GotoTag=Angle
  From4 : From  Commented=on  GotoTag=Velocity
  From5 : From  Commented=on  GotoTag=Velocity
  Gain : Gain  Gain=-1
  Gain1 : Gain  Gain=-1
  Gain5 : Gain  Gain=-1/2
  Gain7 : Gain  Gain=-1/2
  Hit Crossing1 : HitCross  HitCrossingDirection=rising
  Hit Crossing2 : HitCross  HitCrossingDirection=falling
  Hit Crossing3 : HitCross  HitCrossingDirection=rising
  Hit Crossing4 : HitCross  HitCrossingDirection=falling
  IsNaN : RelationalOperator  Operator=isNaN  OutDataTypeStr=boolean  RndMeth=Simplest  InputSameDT=off
  Memory : Memory
  Saturation : Saturate  UpperLimit=10  LowerLimit=-10
  Subsystem : Subsystem
  Subsystem1 : Subsystem
  Subsystem2 : Subsystem
  Subsystem3 : Subsystem
  Subsystem4 : Subsystem  Commented=on
  Subsystem5 : Subsystem  Commented=on
  Subsystem6 : Subsystem  Commented=on
  Subsystem7 : Subsystem  Commented=on
  Sum1 : Sum  Inputs=+-
  Sum2 : Sum  Inputs=-+
  Sum{3..6} (4 alike) : Sum
  Switch : Switch  Criteria=u2 > Threshold  SaturateOnIntegerOverflow=off  InputSameDT=off
  Switch1 : Switch  Criteria=u2 ~= 0  SaturateOnIntegerOverflow=off  InputSameDT=off
  Terminator : Terminator
  Terminator1 : Terminator
  POS SS : Outport
  z(t) : Outport  Port=2
  VEL SS : Outport  Port=3
  wires:
  Hit Crossing2/1 -> Chart/1(ang_max)  "ang_max_trigg_R"
  Subsystem2/1(Angle_max) -> Sum2/2, Sum3/2  "angle_max_R"
  Sum4/1 -> Divide1/1
  Sum3/1 -> Gain5/1
  Subsystem/1(Angle_min) -> Sum2/1, Sum3/1  "angle_min_R"
  Hit Crossing1/1 -> Chart/4(ang_min)  "ang_min_trigg_R"
  Sum2/1 -> Abs1/1
  Sum1/1 -> Abs/1  "(t)_comp"
  Gain5/1 -> Sum4/1  "gamma(t)"
  Abs/1 -> Divide/2
  Divide/1 -> IsNaN/1, Switch/3  "z(t)"
  Memory/1 -> Switch/1
  IsNaN/1 -> Switch/2
  Switch/1 -> Memory/1, Divide1/2, z(t)/1  "z(t)"
  Divide1/1 -> Saturation/1
  Saturation/1 -> POS SS/1
  Clock1/1 -> Subsystem5/2(Clock), Subsystem4/1(Clock)
  Constant/1 -> Switch1/3
  Abs1/1 -> Switch1/2, Switch1/1
  Switch1/1 -> Divide/1
  Clock/1 -> Subsystem7/2(Clock), Subsystem6/2(Clock)
  Hit Crossing4/1 -> Chart/2(vel_min)  "speed_min_trigg_R"
  Subsystem3/1(Vel_min) -> Sum1/2, Sum5/2  "vel_min_R"
  Subsystem1/1(Vel_max) -> Sum1/1, Sum5/1  "Vel_max_R"
  Sum5/1 -> Gain7/1
  Hit Crossing3/1 -> Chart/3(vel_max)  "speed_max_trigg_R"
  Sum6/1 -> VEL SS/1
  Gain7/1 -> Sum6/2  "GAMMA(t)"
  [Velocity] -> Sum6/1
  Chart/1(valid_vel_max) -> Subsystem1/Trigger  "valid_vel_max_R"
  Chart/4(valid_ang_min) -> Gain/1, Subsystem/Trigger  "valid_ang_min_R"
  Chart/3(valid_ang_max) -> Subsystem2/Trigger  "valid_ang_max_R"
  Chart/2(valid_vel_min) -> Gain1/1, Subsystem3/Trigger  "valid_vel_min_R"
  Vel/1 -> [Velocity]
  Angle/1 -> [Angle]
  From5/1 -> Subsystem7/1(Velocity)
  From4/1 -> Subsystem6/1(Velocity)
  From3/1 -> Subsystem5/1(Angle)
  From2/1 -> Subsystem4/2(angle)
  [Angle] -> Hit Crossing4/1, Hit Crossing3/1, Chart/6(angle)
  [Angle] -> Subsystem/1(Angle)
  [Angle] -> Subsystem2/1(angle)
  [Velocity] -> Subsystem1/1(Velocity)
  [Velocity] -> Subsystem3/1(Velocity)
  [Velocity] -> Hit Crossing1/1, Hit Crossing2/1, Chart/5(vel)
  Gain/1 -> Terminator/1  "valid_ang_min_neg_R"
  Gain1/1 -> Terminator1/1  "valid_vel_min_neg_R"
  [Angle] -> Sum4/2

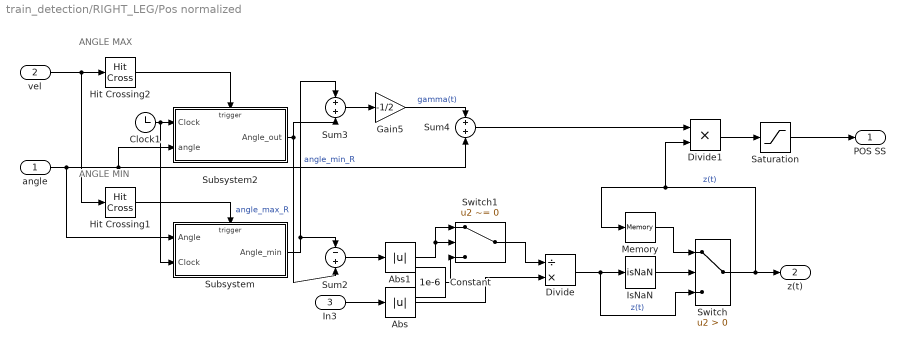
== system train_detection/RIGHT_LEG/Pos normalized ==
  note: ANGLE MIN
  note: ANGLE MAX
  angle : Inport
  vel : Inport  Port=2
  In3 : Inport  Port=3
  Abs : Abs  SaturateOnIntegerOverflow=off
  Abs1 : Abs  SaturateOnIntegerOverflow=off
  Clock1 : Clock
  Constant : Constant  Value=1e-6
  Divide : Product  Inputs=/*
  Divide1 : Product  Inputs=**
  Gain5 : Gain  Gain=-1/2
  Hit Crossing1 : HitCross  HitCrossingDirection=rising
  Hit Crossing2 : HitCross  HitCrossingDirection=falling
  IsNaN : RelationalOperator  Operator=isNaN  OutDataTypeStr=boolean  RndMeth=Simplest  InputSameDT=off
  Memory : Memory
  Saturation : Saturate  UpperLimit=10  LowerLimit=-10
  Subsystem : Subsystem
  Subsystem2 : Subsystem
  Sum2 : Sum  Inputs=-+
  Sum3 : Sum
  Sum4 : Sum
  Switch : Switch  Criteria=u2 > Threshold  SaturateOnIntegerOverflow=off  InputSameDT=off
  Switch1 : Switch  Criteria=u2 ~= 0  SaturateOnIntegerOverflow=off  InputSameDT=off
  POS SS : Outport
  z(t) : Outport  Port=2
  wires:
  Hit Crossing2/1 -> Subsystem2/Trigger
  Subsystem2/1(Angle_out) -> Sum3/2, Sum2/2  "angle_max_R"
  Sum4/1 -> Divide1/1
  Sum3/1 -> Gain5/1
  Subsystem/1(Angle_min) -> Sum3/1, Sum2/1  "angle_min_R"
  Hit Crossing1/1 -> Subsystem/Trigger
  angle/1 -> Subsystem2/2(angle), Sum4/2, Subsystem/1(Angle)
  vel/1 -> Hit Crossing1/1, Hit Crossing2/1
  Sum2/1 -> Abs1/1
  In3/1 -> Abs/1
  Gain5/1 -> Sum4/1  "gamma(t)"
  Abs1/1 -> Switch1/2, Switch1/1
  Abs/1 -> Divide/2
  Divide/1 -> IsNaN/1, Switch/3  "z(t)"
  Memory/1 -> Switch/1
  IsNaN/1 -> Switch/2
  Switch/1 -> Memory/1, Divide1/2, z(t)/1  "z(t)"
  Divide1/1 -> Saturation/1
  Saturation/1 -> POS SS/1
  Clock1/1 -> Subsystem2/1(Clock), Subsystem/2(Clock)
  Switch1/1 -> Divide/1
  Constant/1 -> Switch1/3

== system train_detection/RIGHT_LEG/STOP CONDITION ==
  position : Inport
  speed : Inport  Port=2
  Constant : Constant
  Constant1 : Constant  Value=0
  Sqrt : Sqrt
  Square : Math  Operator=square
  Square1 : Math  Operator=square
  Sum : Sum
  Switch3 : Switch  Criteria=u2 > Threshold  Threshold=0.3  SaturateOnIntegerOverflow=off  InputSameDT=off
  Check : Outport
  Walking frequency : Outport  Port=2
  wires:
  position/1 -> Square/1  "θ"
  speed/1 -> Square1/1  "θ_dot"
  Square/1 -> Sum/1
  Square1/1 -> Sum/2
  Sum/1 -> Sqrt/1
  Constant/1 -> Switch3/1
  Constant1/1 -> Switch3/3
  Sqrt/1 -> Switch3/2, Walking frequency/1
  Switch3/1 -> Check/1

== system train_detection/RIGHT_LEG/Vel normalized ==
  note: SPEED MAX
  note: SPEED MIN
  Ang : Inport
  Velocity : Inport  Port=2
  Clock : Clock
  Gain7 : Gain  Gain=-1/2
  Hit Crossing3 : HitCross  HitCrossingDirection=rising
  Hit Crossing4 : HitCross  HitCrossingDirection=falling
  Subsystem1 : Subsystem
  Subsystem3 : Subsystem
  Sum1 : Sum  Inputs=+-
  Sum5 : Sum
  Sum6 : Sum
  Out1 : Outport
  VEL SS : Outport  Port=2
  wires:
  Sum5/1 -> Gain7/1
  Subsystem1/1(Vel_max) -> Sum1/1, Sum5/1  "vel_max_R"
  Sum1/1 -> Out1/1
  Subsystem3/1(Vel_min) -> Sum1/2, Sum5/2  "vel_min_R"
  Ang/1 -> Hit Crossing4/1, Hit Crossing3/1
  Gain7/1 -> Sum6/2  "GAMMA(t)"
  Sum6/1 -> VEL SS/1
  Velocity/1 -> Sum6/1, Subsystem1/1(Velocity), Subsystem3/1(Velocity)
  Hit Crossing3/1 -> Subsystem1/Trigger  "Angle_0_pos_R"
  Hit Crossing4/1 -> Subsystem3/Trigger  "Angle_0_neg_R"
  Clock/1 -> Subsystem1/2(Clock), Subsystem3/2(Clock)

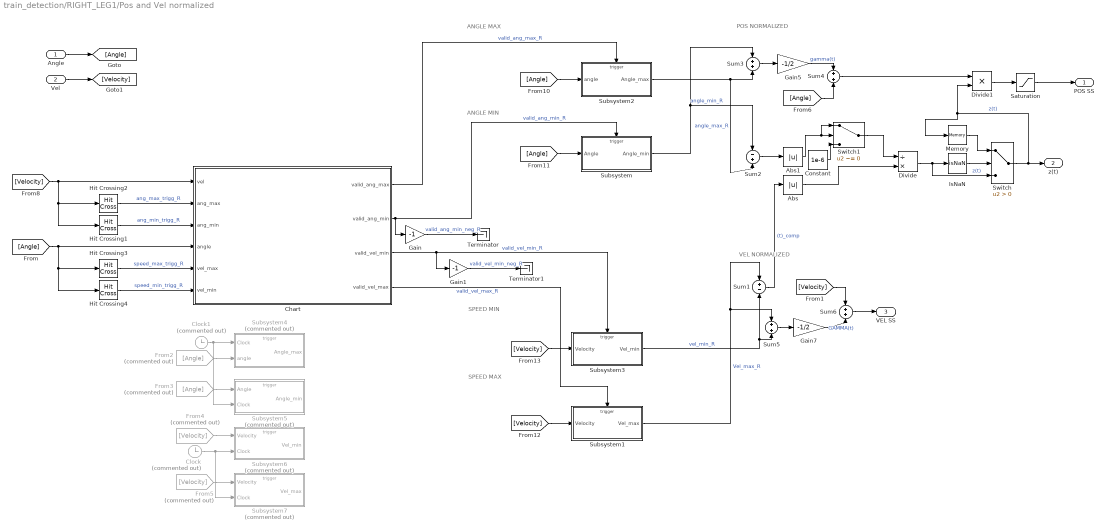
== system train_detection/RIGHT_LEG1/Pos and Vel normalized ==
  note: ANGLE MIN
  note: ANGLE MAX
  note: SPEED MAX
  note: SPEED MIN
  note: POS NORMALIZED
  note: VEL NORMALIZED
  Angle : Inport
  Vel : Inport  Port=2
  Abs : Abs  SaturateOnIntegerOverflow=off
  Abs1 : Abs  SaturateOnIntegerOverflow=off
  Chart : Stateflow chart  TreatAsAtomicUnit=on
      settings: PortSchema="{\"entries\":[{\"content\":{\"sides\":[{\"content\":{\"connectorIds\":[\"In5\",\"In1\",\"In4\",\"In6\",\"In3\",\"In2\"]},\"type\":\"ConnectorPlacement.EquallySpacedRectSide\",\"uuid\":\"1b4e9464-0c1b-4aef-9691-eb83c0a92a72\"},{\"content\":{\"connectorIds\":[\"Out3\",\"Out4\",\"Out2\",\"Out1\"],\"side\":\"RIGHT\"},\"type\":\"ConnectorPlacement.EquallySpacedRectSide\",\"uuid\":\"791196f6-4c97-40a1-8015-a03f83b94293\"},{\"content\":{\"side\":\"TOP\"},\"type\":\"ConnectorPlacement.EquallySpacedRectSide\",\"uuid\":\"116d3fb6-be2c-4be4-86cc-df9779b501c6\"}]},\"type\":\"ConnectorPlacement.EquallySpacedConnector\",\"uuid\":\"13d090b2-a2d1-429a-b321-7320a6f027c7\"}],\"packageUris\":[\"http://schema.mathworks.com/mf0/Connector/R2020b\"],\"version\":\"1.0\"}"
  Clock : Clock  Commented=on
  Clock1 : Clock  Commented=on
  Constant : Constant  Value=1e-6
  Divide : Product  Inputs=/*
  Divide1 : Product  Inputs=**
  From2 : From  Commented=on  GotoTag=Angle
  From3 : From  Commented=on  GotoTag=Angle
  From4 : From  Commented=on  GotoTag=Velocity
  From5 : From  Commented=on  GotoTag=Velocity
  Gain : Gain  Gain=-1
  Gain1 : Gain  Gain=-1
  Gain5 : Gain  Gain=-1/2
  Gain7 : Gain  Gain=-1/2
  Hit Crossing1 : HitCross  HitCrossingDirection=rising
  Hit Crossing2 : HitCross  HitCrossingDirection=falling
  Hit Crossing3 : HitCross  HitCrossingDirection=rising
  Hit Crossing4 : HitCross  HitCrossingDirection=falling
  IsNaN : RelationalOperator  Operator=isNaN  OutDataTypeStr=boolean  RndMeth=Simplest  InputSameDT=off
  Memory : Memory
  Saturation : Saturate  UpperLimit=10  LowerLimit=-10
  Subsystem : Subsystem
  Subsystem1 : Subsystem
  Subsystem2 : Subsystem
  Subsystem3 : Subsystem
  Subsystem4 : Subsystem  Commented=on
  Subsystem5 : Subsystem  Commented=on
  Subsystem6 : Subsystem  Commented=on
  Subsystem7 : Subsystem  Commented=on
  Sum1 : Sum  Inputs=+-
  Sum2 : Sum  Inputs=-+
  Sum{3..6} (4 alike) : Sum
  Switch : Switch  Criteria=u2 > Threshold  SaturateOnIntegerOverflow=off  InputSameDT=off
  Switch1 : Switch  Criteria=u2 ~= 0  SaturateOnIntegerOverflow=off  InputSameDT=off
  Terminator : Terminator
  Terminator1 : Terminator
  POS SS : Outport
  z(t) : Outport  Port=2
  VEL SS : Outport  Port=3
  wires:
  Hit Crossing2/1 -> Chart/1(ang_max)  "ang_max_trigg_R"
  Subsystem2/1(Angle_max) -> Sum2/2, Sum3/2  "angle_max_R"
  Sum4/1 -> Divide1/1
  Sum3/1 -> Gain5/1
  Subsystem/1(Angle_min) -> Sum2/1, Sum3/1  "angle_min_R"
  Hit Crossing1/1 -> Chart/4(ang_min)  "ang_min_trigg_R"
  Sum2/1 -> Abs1/1
  Sum1/1 -> Abs/1  "(t)_comp"
  Gain5/1 -> Sum4/1  "gamma(t)"
  Abs/1 -> Divide/2
  Divide/1 -> IsNaN/1, Switch/3  "z(t)"
  Memory/1 -> Switch/1
  IsNaN/1 -> Switch/2
  Switch/1 -> Memory/1, Divide1/2, z(t)/1  "z(t)"
  Divide1/1 -> Saturation/1
  Saturation/1 -> POS SS/1
  Clock1/1 -> Subsystem5/2(Clock), Subsystem4/1(Clock)
  Constant/1 -> Switch1/3
  Abs1/1 -> Switch1/2, Switch1/1
  Switch1/1 -> Divide/1
  Clock/1 -> Subsystem7/2(Clock), Subsystem6/2(Clock)
  Hit Crossing4/1 -> Chart/2(vel_min)  "speed_min_trigg_R"
  Subsystem3/1(Vel_min) -> Sum1/2, Sum5/2  "vel_min_R"
  Subsystem1/1(Vel_max) -> Sum1/1, Sum5/1  "Vel_max_R"
  Sum5/1 -> Gain7/1
  Hit Crossing3/1 -> Chart/3(vel_max)  "speed_max_trigg_R"
  Sum6/1 -> VEL SS/1
  Gain7/1 -> Sum6/2  "GAMMA(t)"
  [Velocity] -> Sum6/1
  Chart/1(valid_vel_max) -> Subsystem1/Trigger  "valid_vel_max_R"
  Chart/4(valid_ang_min) -> Gain/1, Subsystem/Trigger  "valid_ang_min_R"
  Chart/3(valid_ang_max) -> Subsystem2/Trigger  "valid_ang_max_R"
  Chart/2(valid_vel_min) -> Gain1/1, Subsystem3/Trigger  "valid_vel_min_R"
  Vel/1 -> [Velocity]
  Angle/1 -> [Angle]
  From5/1 -> Subsystem7/1(Velocity)
  From4/1 -> Subsystem6/1(Velocity)
  From3/1 -> Subsystem5/1(Angle)
  From2/1 -> Subsystem4/2(angle)
  [Angle] -> Hit Crossing4/1, Hit Crossing3/1, Chart/6(angle)
  [Angle] -> Subsystem/1(Angle)
  [Angle] -> Subsystem2/1(angle)
  [Velocity] -> Subsystem1/1(Velocity)
  [Velocity] -> Subsystem3/1(Velocity)
  [Velocity] -> Hit Crossing1/1, Hit Crossing2/1, Chart/5(vel)
  Gain/1 -> Terminator/1  "valid_ang_min_neg_R"
  Gain1/1 -> Terminator1/1  "valid_vel_min_neg_R"
  [Angle] -> Sum4/2

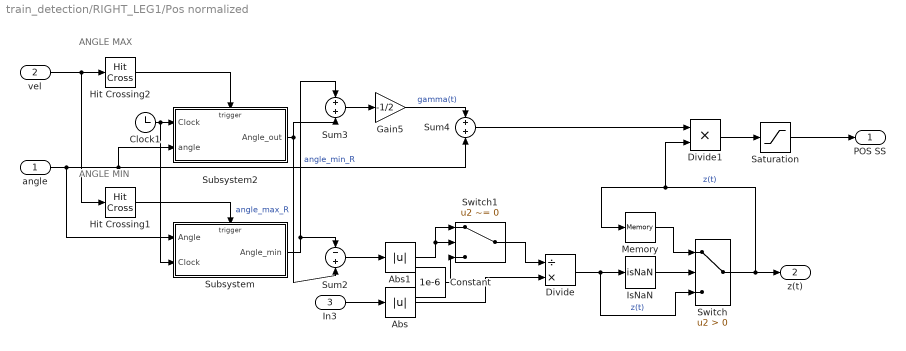
== system train_detection/RIGHT_LEG1/Pos normalized ==
  note: ANGLE MIN
  note: ANGLE MAX
  angle : Inport
  vel : Inport  Port=2
  In3 : Inport  Port=3
  Abs : Abs  SaturateOnIntegerOverflow=off
  Abs1 : Abs  SaturateOnIntegerOverflow=off
  Clock1 : Clock
  Constant : Constant  Value=1e-6
  Divide : Product  Inputs=/*
  Divide1 : Product  Inputs=**
  Gain5 : Gain  Gain=-1/2
  Hit Crossing1 : HitCross  HitCrossingDirection=rising
  Hit Crossing2 : HitCross  HitCrossingDirection=falling
  IsNaN : RelationalOperator  Operator=isNaN  OutDataTypeStr=boolean  RndMeth=Simplest  InputSameDT=off
  Memory : Memory
  Saturation : Saturate  UpperLimit=10  LowerLimit=-10
  Subsystem : Subsystem
  Subsystem2 : Subsystem
  Sum2 : Sum  Inputs=-+
  Sum3 : Sum
  Sum4 : Sum
  Switch : Switch  Criteria=u2 > Threshold  SaturateOnIntegerOverflow=off  InputSameDT=off
  Switch1 : Switch  Criteria=u2 ~= 0  SaturateOnIntegerOverflow=off  InputSameDT=off
  POS SS : Outport
  z(t) : Outport  Port=2
  wires:
  Hit Crossing2/1 -> Subsystem2/Trigger
  Subsystem2/1(Angle_out) -> Sum3/2, Sum2/2  "angle_max_R"
  Sum4/1 -> Divide1/1
  Sum3/1 -> Gain5/1
  Subsystem/1(Angle_min) -> Sum3/1, Sum2/1  "angle_min_R"
  Hit Crossing1/1 -> Subsystem/Trigger
  angle/1 -> Subsystem2/2(angle), Sum4/2, Subsystem/1(Angle)
  vel/1 -> Hit Crossing1/1, Hit Crossing2/1
  Sum2/1 -> Abs1/1
  In3/1 -> Abs/1
  Gain5/1 -> Sum4/1  "gamma(t)"
  Abs1/1 -> Switch1/2, Switch1/1
  Abs/1 -> Divide/2
  Divide/1 -> IsNaN/1, Switch/3  "z(t)"
  Memory/1 -> Switch/1
  IsNaN/1 -> Switch/2
  Switch/1 -> Memory/1, Divide1/2, z(t)/1  "z(t)"
  Divide1/1 -> Saturation/1
  Saturation/1 -> POS SS/1
  Clock1/1 -> Subsystem2/1(Clock), Subsystem/2(Clock)
  Switch1/1 -> Divide/1
  Constant/1 -> Switch1/3

== system train_detection/RIGHT_LEG1/STOP CONDITION ==
  position : Inport
  speed : Inport  Port=2
  Constant : Constant
  Constant1 : Constant  Value=0
  Sqrt : Sqrt
  Square : Math  Operator=square
  Square1 : Math  Operator=square
  Sum : Sum
  Switch3 : Switch  Criteria=u2 > Threshold  Threshold=0.3  SaturateOnIntegerOverflow=off  InputSameDT=off
  Check : Outport
  Walking frequency : Outport  Port=2
  wires:
  position/1 -> Square/1  "θ"
  speed/1 -> Square1/1  "θ_dot"
  Square/1 -> Sum/1
  Square1/1 -> Sum/2
  Sum/1 -> Sqrt/1
  Constant/1 -> Switch3/1
  Constant1/1 -> Switch3/3
  Sqrt/1 -> Switch3/2, Walking frequency/1
  Switch3/1 -> Check/1

== system train_detection/RIGHT_LEG1/Vel normalized ==
  note: SPEED MAX
  note: SPEED MIN
  Ang : Inport
  Velocity : Inport  Port=2
  Clock : Clock
  Gain7 : Gain  Gain=-1/2
  Hit Crossing3 : HitCross  HitCrossingDirection=rising
  Hit Crossing4 : HitCross  HitCrossingDirection=falling
  Subsystem1 : Subsystem
  Subsystem3 : Subsystem
  Sum1 : Sum  Inputs=+-
  Sum5 : Sum
  Sum6 : Sum
  Out1 : Outport
  VEL SS : Outport  Port=2
  wires:
  Sum5/1 -> Gain7/1
  Subsystem1/1(Vel_max) -> Sum1/1, Sum5/1  "vel_max_R"
  Sum1/1 -> Out1/1
  Subsystem3/1(Vel_min) -> Sum1/2, Sum5/2  "vel_min_R"
  Ang/1 -> Hit Crossing4/1, Hit Crossing3/1
  Gain7/1 -> Sum6/2  "GAMMA(t)"
  Sum6/1 -> VEL SS/1
  Velocity/1 -> Sum6/1, Subsystem1/1(Velocity), Subsystem3/1(Velocity)
  Hit Crossing3/1 -> Subsystem1/Trigger  "Angle_0_pos_R"
  Hit Crossing4/1 -> Subsystem3/Trigger  "Angle_0_neg_R"
  Clock/1 -> Subsystem1/2(Clock), Subsystem3/2(Clock)

== system train_detection/LEFT LEG/Pos and Vel normalized/Subsystem ==
  Angle : Inport
  Trigger : TriggerPort  VariantControl=Variant  PortDimensions=1
  Angle_min : Outport
  wires:
  Angle/1 -> Angle_min/1

== system train_detection/LEFT LEG/Pos and Vel normalized/Subsystem1 ==
  Velocity : Inport
  Trigger : TriggerPort  VariantControl=Variant  PortDimensions=1
  Vel_max : Outport
  wires:
  Velocity/1 -> Vel_max/1

== system train_detection/LEFT LEG/Pos and Vel normalized/Subsystem2 ==
  angle : Inport
  Trigger : TriggerPort  VariantControl=Variant  PortDimensions=1
  Angle_max : Outport
  wires:
  angle/1 -> Angle_max/1

== system train_detection/LEFT LEG/Pos and Vel normalized/Subsystem3 ==
  Velocity : Inport
  Trigger : TriggerPort  VariantControl=Variant  PortDimensions=1
  Vel_min : Outport
  wires:
  Velocity/1 -> Vel_min/1

== system train_detection/LEFT LEG/Pos and Vel normalized/Subsystem4 ==
  Clock : Inport
  angle : Inport  Port=2
  Trigger : TriggerPort  VariantControl=Variant  PortDimensions=1
  If : If  ShowElse=off
  If Action Subsystem : Subsystem  TreatAsAtomicUnit=on
  Angle_max : Outport
  wires:
  If/1 -> If Action Subsystem/Action
  angle/1 -> If Action Subsystem/2(angle), If/1
  If Action Subsystem/1(Angle_max) -> Angle_max/1  "angle_max"
  Clock/1 -> If Action Subsystem/1(Clock)  "clock"

== system train_detection/LEFT LEG/Pos and Vel normalized/Subsystem5 ==
  Angle : Inport
  Clock : Inport  Port=2
  Trigger : TriggerPort  VariantControl=Variant  PortDimensions=1
  If : If  IfExpression=u1 < 0  ShowElse=off
  If Action Subsystem : Subsystem  TreatAsAtomicUnit=on
  Angle_min : Outport
  wires:
  If/1 -> If Action Subsystem/Action
  Angle/1 -> If Action Subsystem/1(Angle), If/1
  If Action Subsystem/1(Angle_min) -> Angle_min/1  "angle_min"
  Clock/1 -> If Action Subsystem/2(Clock)  "clock"

== system train_detection/LEFT LEG/Pos and Vel normalized/Subsystem6 ==
  Velocity : Inport
  Clock : Inport  Port=2
  Trigger : TriggerPort  VariantControl=Variant  PortDimensions=1
  If : If  IfExpression=u1 < 0  ShowElse=off
  If Action Subsystem : Subsystem  TreatAsAtomicUnit=on
  Vel_min : Outport
  wires:
  If Action Subsystem/1(Vel_min) -> Vel_min/1  "vel_min"
  If/1 -> If Action Subsystem/Action
  Velocity/1 -> If Action Subsystem/1(Velocity), If/1
  Clock/1 -> If Action Subsystem/2(Clock)  "clock"

== system train_detection/LEFT LEG/Pos and Vel normalized/Subsystem7 ==
  Velocity : Inport
  Clock : Inport  Port=2
  Trigger : TriggerPort  VariantControl=Variant  PortDimensions=1
  If : If  ShowElse=off
  If Action Subsystem : Subsystem  TreatAsAtomicUnit=on
  Vel_max : Outport
  wires:
  If/1 -> If Action Subsystem/Action
  Velocity/1 -> If Action Subsystem/1(Velocity), If/1
  Clock/1 -> If Action Subsystem/2(Clock)  "clock"
  If Action Subsystem/1(Vel_max) -> Vel_max/1  "vel_max"

== system train_detection/LEFT LEG1/Pos and Vel normalized/Subsystem ==
  Angle : Inport
  Trigger : TriggerPort  VariantControl=Variant  PortDimensions=1
  Angle_min : Outport
  wires:
  Angle/1 -> Angle_min/1

== system train_detection/LEFT LEG1/Pos and Vel normalized/Subsystem1 ==
  Velocity : Inport
  Trigger : TriggerPort  VariantControl=Variant  PortDimensions=1
  Vel_max : Outport
  wires:
  Velocity/1 -> Vel_max/1

== system train_detection/LEFT LEG1/Pos and Vel normalized/Subsystem2 ==
  angle : Inport
  Trigger : TriggerPort  VariantControl=Variant  PortDimensions=1
  Angle_max : Outport
  wires:
  angle/1 -> Angle_max/1

== system train_detection/LEFT LEG1/Pos and Vel normalized/Subsystem3 ==
  Velocity : Inport
  Trigger : TriggerPort  VariantControl=Variant  PortDimensions=1
  Vel_min : Outport
  wires:
  Velocity/1 -> Vel_min/1

== system train_detection/LEFT LEG1/Pos and Vel normalized/Subsystem4 ==
  Clock : Inport
  angle : Inport  Port=2
  Trigger : TriggerPort  VariantControl=Variant  PortDimensions=1
  If : If  ShowElse=off
  If Action Subsystem : Subsystem  TreatAsAtomicUnit=on
  Angle_max : Outport
  wires:
  If/1 -> If Action Subsystem/Action
  angle/1 -> If Action Subsystem/2(angle), If/1
  If Action Subsystem/1(Angle_max) -> Angle_max/1  "angle_max"
  Clock/1 -> If Action Subsystem/1(Clock)  "clock"

== system train_detection/LEFT LEG1/Pos and Vel normalized/Subsystem5 ==
  Angle : Inport
  Clock : Inport  Port=2
  Trigger : TriggerPort  VariantControl=Variant  PortDimensions=1
  If : If  IfExpression=u1 < 0  ShowElse=off
  If Action Subsystem : Subsystem  TreatAsAtomicUnit=on
  Angle_min : Outport
  wires:
  If/1 -> If Action Subsystem/Action
  Angle/1 -> If Action Subsystem/1(Angle), If/1
  If Action Subsystem/1(Angle_min) -> Angle_min/1  "angle_min"
  Clock/1 -> If Action Subsystem/2(Clock)  "clock"

== system train_detection/LEFT LEG1/Pos and Vel normalized/Subsystem6 ==
  Velocity : Inport
  Clock : Inport  Port=2
  Trigger : TriggerPort  VariantControl=Variant  PortDimensions=1
  If : If  IfExpression=u1 < 0  ShowElse=off
  If Action Subsystem : Subsystem  TreatAsAtomicUnit=on
  Vel_min : Outport
  wires:
  If Action Subsystem/1(Vel_min) -> Vel_min/1  "vel_min"
  If/1 -> If Action Subsystem/Action
  Velocity/1 -> If Action Subsystem/1(Velocity), If/1
  Clock/1 -> If Action Subsystem/2(Clock)  "clock"

== system train_detection/LEFT LEG1/Pos and Vel normalized/Subsystem7 ==
  Velocity : Inport
  Clock : Inport  Port=2
  Trigger : TriggerPort  VariantControl=Variant  PortDimensions=1
  If : If  ShowElse=off
  If Action Subsystem : Subsystem  TreatAsAtomicUnit=on
  Vel_max : Outport
  wires:
  If/1 -> If Action Subsystem/Action
  Velocity/1 -> If Action Subsystem/1(Velocity), If/1
  Clock/1 -> If Action Subsystem/2(Clock)  "clock"
  If Action Subsystem/1(Vel_max) -> Vel_max/1  "vel_max"
